simulink library "EasyGen3500_GensetSignalScaling_lib"  (Simulink 8.1)
settings: Solver=ode45  StartTime=0.0  StopTime=10.0  RelTol=1e-3
undefined symbols (not defined in the file): ph, Ts
libraries: rteventslib x4
settings Model: Creator=RE25624  LastModifiedBy=RE25624

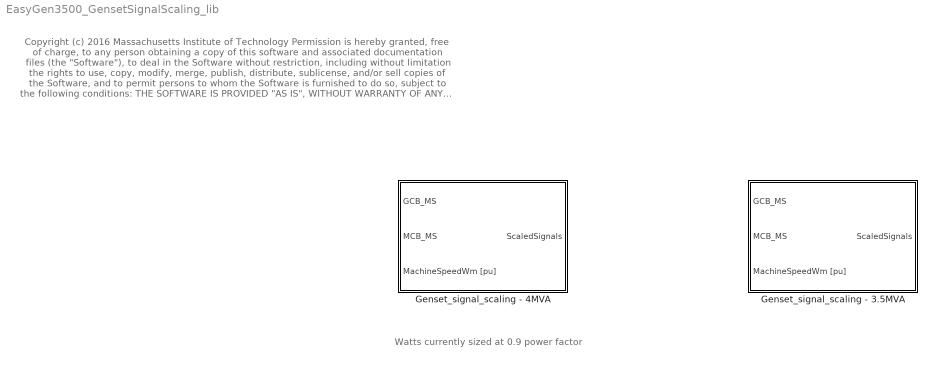
== system EasyGen3500_GensetSignalScaling_lib ==
  note: Watts currently sized at 0.9 power factor
  note: Copyright (c) 2016 Massachusetts Institute of Technology
      | Permission is hereby granted, free of charge, to any person obtaining a copy of this software and associated documentation files (the "Software"), to deal
      | in the Software without restriction, including without limitation the rights to use, copy, modify, merge, publish, distribute, sublicense, and/or sell copies of the
      | Software, and to permit persons to whom the Software is furnished to do so, subject to the following conditions:
      |
      | THE SOFTWARE IS PROVIDED "AS IS", WITHOUT WARRANTY OF ANY KIND, EXPRESS OR IMPLIED, INCLUDING BUT NOT LIMITED TO THE
      | WARRANTIES OF MERCHANTABILITY, FITNESS FOR A PARTICULAR PURPOSE AND NONINFRINGEMENT. IN NO EVENT SHALL THE AUTHORS
      | OR COPYRIGHT HOLDERS BE LIABLE FOR ANY CLAIM, DAMAGES OR OTHER LIABILITY, WHETHER IN AN ACTION OF CONTRACT, TORT OR
      | OTHERWISE, ARISING FROM, OUT OF OR IN CONNECTION WITH THE SOFTWARE OR THE USE OR OTHER DEALINGS IN THE SOFTWARE
  Genset_signal_scaling - 3.5MVA : Subsystem  mask(Genset Signal Scaling for Opal-RT/Woodward){Vpk_mcb=11268, watt_mcb=3150000, Vpk_gcb=11268, watt_gcb=3150000, rated_rpm=1800, wm_noise_bias=0.02}
      mask prompts: Vpk_mcb "MCB Nominal Voltage [Vpk]"; watt_mcb "MCB Watts [W]"; Vpk_gcb "GCB Nominal Voltage [ Vpk]"; watt_gcb "GCB Watts [W]"; rated_rpm "Machine Rated Speed [RPM]"; wm_noise_bias "Speed Noise Bias [0-1]"
      mask help:
      | Scaling for voltages:
      | For 120 => 12Vout / 170Vpk
      | For 480 => 12Vout / 391Vpk
      | For 13.8kv => 12Vout / 11268Vpk
      |
      | Scaling for currents - used in the 1 MVA genset:
      | 15Vout / ( 900000W / 391Vpk)
      |
      | Scaling for currents - used in the 3.5 MVA NG/CHP:
      | 15Vout / ( 3150000W / 11268Vpk)
      | - Current scale factors chosen to match easYgen settings for 3.5 MVA gas engine CT ratio of 1500/x made on 20160508
  Genset_signal_scaling - 4MVA : Subsystem  mask(Genset Signal Scaling for Opal-RT/Woodward){Vpk_mcb=11268, watt_mcb=3600000, Vpk_gcb=11268, watt_gcb=3600000, rated_rpm=1800, wm_noise_bias=0.02}
      mask prompts: Vpk_mcb "MCB Nominal Voltage [Vpk]"; watt_mcb "MCB Watts [W]"; Vpk_gcb "GCB Nominal Voltage [ Vpk]"; watt_gcb "GCB Watts [W]"; rated_rpm "Machine Rated Speed [RPM]"; wm_noise_bias "Speed Noise Bias [0-1]"
      mask help:
      | Scaling for voltages:
      | For 120 => 12Vout / 170Vpk
      | For 480 => 12Vout / 391Vpk
      | For 13.8kv => 12Vout / 11268Vpk
      |
      | Scaling for currents - used in the 1 MVA genset:
      | 15Vout / ( 900000W / 391Vpk)
      |
      | Scaling for currents - used in the 3.5 MVA NG/CHP:
      | 15Vout / ( 3150000W / 11268Vpk)
      | - Current scale factors chosen to match easYgen settings for 3.5 MVA gas engine CT ratio of 1500/x made on 20160508

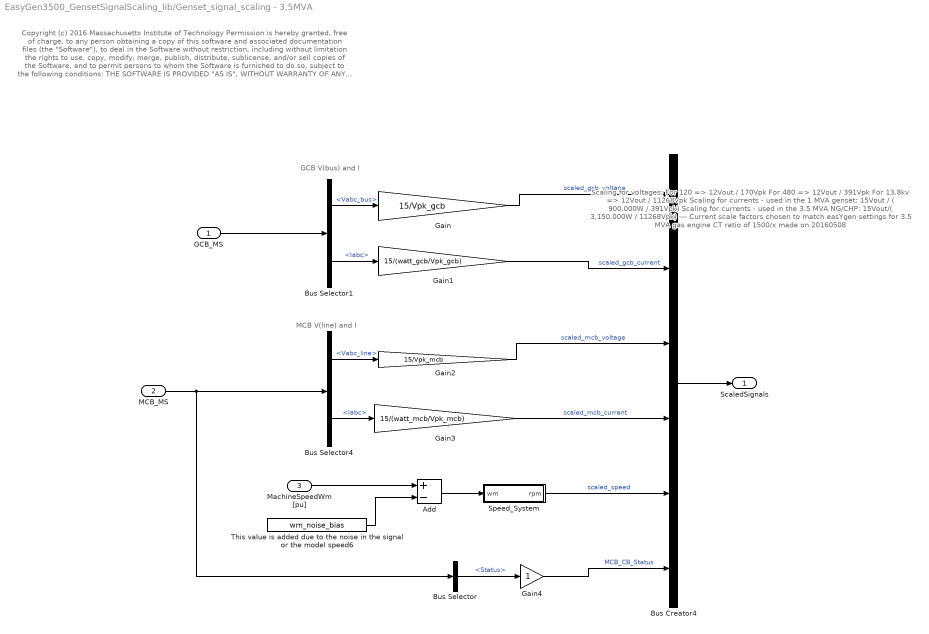
== system EasyGen3500_GensetSignalScaling_lib/Genset_signal_scaling - 3.5MVA ==
  note: Copyright (c) 2016 Massachusetts Institute of Technology
      | Permission is hereby granted, free of charge, to any person obtaining a copy of this software and associated documentation files (the "Software"), to deal
      | in the Software without restriction, including without limitation the rights to use, copy, modify, merge, publish, distribute, sublicense, and/or sell copies of the
      | Software, and to permit persons to whom the Software is furnished to do so, subject to the following conditions:
      |
      | THE SOFTWARE IS PROVIDED "AS IS", WITHOUT WARRANTY OF ANY KIND, EXPRESS OR IMPLIED, INCLUDING BUT NOT LIMITED TO THE
      | WARRANTIES OF MERCHANTABILITY, FITNESS FOR A PARTICULAR PURPOSE AND NONINFRINGEMENT. IN NO EVENT SHALL THE AUTHORS
      | OR COPYRIGHT HOLDERS BE LIABLE FOR ANY CLAIM, DAMAGES OR OTHER LIABILITY, WHETHER IN AN ACTION OF CONTRACT, TORT OR
      | OTHERWISE, ARISING FROM, OUT OF OR IN CONNECTION WITH THE SOFTWARE OR THE USE OR OTHER DEALINGS IN THE SOFTWARE
  note: Scaling for voltages:
      | For 120 => 12Vout / 170Vpk
      | For 480 => 12Vout / 391Vpk
      | For 13.8kv => 12Vout / 11268Vpk
      |
      | Scaling for currents - used in the 1 MVA genset:
      | 15Vout / ( 900,000W / 391Vpk)
      |
      | Scaling for currents - used in the 3.5 MVA NG/CHP:
      | 15Vout/( 3,150,000W / 11268Vpk)
      | --- Current scale factors chosen to match easYgen settings for 3.5 MVA gas engine CT ratio of 1500/x made on 20160508
  note: MCB V(line) and I
  note: GCB V(bus) and I
  GCB_MS : Inport
  MCB_MS : Inport  Port=2
  MachineSpeedWm [pu] : Inport  Port=3
  Add : Sum  Inputs=+-
  Bus Creator4 : BusCreator  Inputs=6
  Bus Selector : BusSelector  OutputSignals=Status
  Bus Selector1 : BusSelector  OutputSignals=Vabc_bus,Iabc
  Bus Selector4 : BusSelector  OutputSignals=Vabc_line,Iabc
  Gain : Gain  Gain=15/Vpk_gcb
  Gain1 : Gain  Gain=15/(watt_gcb/Vpk_gcb)
  Gain2 : Gain  Gain=15/Vpk_mcb
  Gain3 : Gain  Gain=15/(watt_mcb/Vpk_mcb)
  Gain4 : Gain
  Speed_System : Subsystem  mask{rated_rpm=rated_rpm}
      mask prompts: rated_rpm "Machine Rated Speed [RPM]"
  This value is added due to the noise in the signal or the model speed6 : Constant  Value=wm_noise_bias
  ScaledSignals : Outport
  wires:
  Bus Selector/1 -> Gain4/1  "<Status>"
  Gain4/1 -> Bus Creator4/6  "MCB_CB_Status"
  Gain/1 -> Bus Creator4/1  "scaled_gcb_voltage"
  Gain1/1 -> Bus Creator4/2  "scaled_gcb_current"
  Speed_System/1(rpm) -> Bus Creator4/5  "scaled_speed"
  Gain2/1 -> Bus Creator4/3  "scaled_mcb_voltage"
  Bus Creator4/1 -> ScaledSignals/1
  Bus Selector4/1 -> Gain2/1  "<Vabc_line>"
  Bus Selector4/2 -> Gain3/1  "<Iabc>"
  Gain3/1 -> Bus Creator4/4  "scaled_mcb_current"
  Bus Selector1/2 -> Gain1/1  "<Iabc>"
  Bus Selector1/1 -> Gain/1  "<Vabc_bus>"
  Add/1 -> Speed_System/1(wm)
  MCB_MS/1 -> Bus Selector/1, Bus Selector4/1
  GCB_MS/1 -> Bus Selector1/1
  MachineSpeedWm [pu]/1 -> Add/1
  This value is added due to the noise in the signal or the model speed6/1 -> Add/2

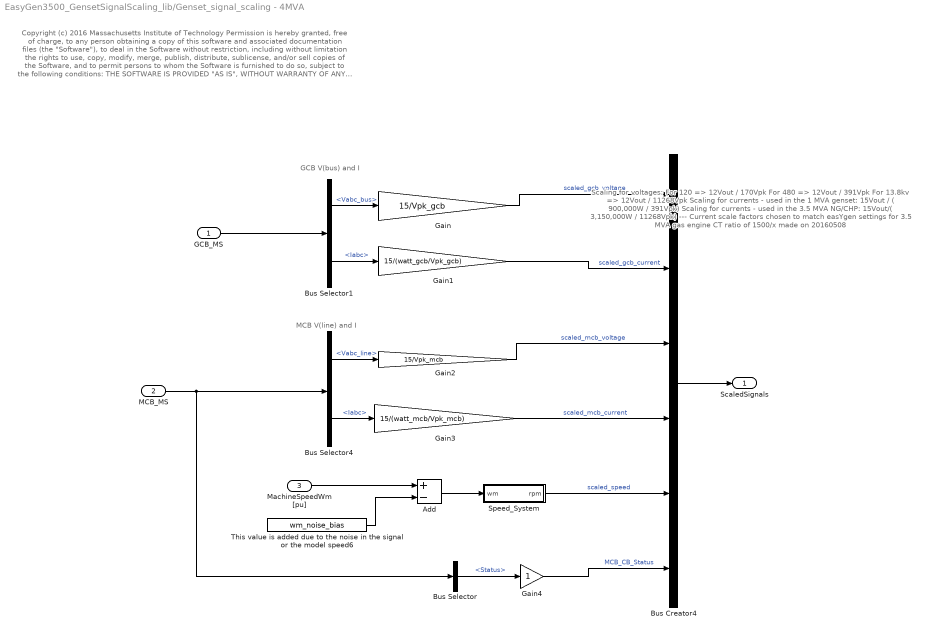
== system EasyGen3500_GensetSignalScaling_lib/Genset_signal_scaling - 4MVA ==
  note: GCB V(bus) and I
  note: MCB V(line) and I
  note: Scaling for voltages:
      | For 120 => 12Vout / 170Vpk
      | For 480 => 12Vout / 391Vpk
      | For 13.8kv => 12Vout / 11268Vpk
      |
      | Scaling for currents - used in the 1 MVA genset:
      | 15Vout / ( 900,000W / 391Vpk)
      |
      | Scaling for currents - used in the 3.5 MVA NG/CHP:
      | 15Vout/( 3,150,000W / 11268Vpk)
      | --- Current scale factors chosen to match easYgen settings for 3.5 MVA gas engine CT ratio of 1500/x made on 20160508
  note: Copyright (c) 2016 Massachusetts Institute of Technology
      | Permission is hereby granted, free of charge, to any person obtaining a copy of this software and associated documentation files (the "Software"), to deal
      | in the Software without restriction, including without limitation the rights to use, copy, modify, merge, publish, distribute, sublicense, and/or sell copies of the
      | Software, and to permit persons to whom the Software is furnished to do so, subject to the following conditions:
      |
      | THE SOFTWARE IS PROVIDED "AS IS", WITHOUT WARRANTY OF ANY KIND, EXPRESS OR IMPLIED, INCLUDING BUT NOT LIMITED TO THE
      | WARRANTIES OF MERCHANTABILITY, FITNESS FOR A PARTICULAR PURPOSE AND NONINFRINGEMENT. IN NO EVENT SHALL THE AUTHORS
      | OR COPYRIGHT HOLDERS BE LIABLE FOR ANY CLAIM, DAMAGES OR OTHER LIABILITY, WHETHER IN AN ACTION OF CONTRACT, TORT OR
      | OTHERWISE, ARISING FROM, OUT OF OR IN CONNECTION WITH THE SOFTWARE OR THE USE OR OTHER DEALINGS IN THE SOFTWARE
  GCB_MS : Inport
  MCB_MS : Inport  Port=2
  MachineSpeedWm [pu] : Inport  Port=3
  Add : Sum  Inputs=+-
  Bus Creator4 : BusCreator  Inputs=6
  Bus Selector : BusSelector  OutputSignals=Status
  Bus Selector1 : BusSelector  OutputSignals=Vabc_bus,Iabc
  Bus Selector4 : BusSelector  OutputSignals=Vabc_line,Iabc
  Gain : Gain  Gain=15/Vpk_gcb
  Gain1 : Gain  Gain=15/(watt_gcb/Vpk_gcb)
  Gain2 : Gain  Gain=15/Vpk_mcb
  Gain3 : Gain  Gain=15/(watt_mcb/Vpk_mcb)
  Gain4 : Gain
  Speed_System : Subsystem  mask{rated_rpm=rated_rpm}
      mask prompts: rated_rpm "Machine Rated Speed [RPM]"
  This value is added due to the noise in the signal or the model speed6 : Constant  Value=wm_noise_bias
  ScaledSignals : Outport
  wires:
  This value is added due to the noise in the signal or the model speed6/1 -> Add/2
  MachineSpeedWm [pu]/1 -> Add/1
  GCB_MS/1 -> Bus Selector1/1
  MCB_MS/1 -> Bus Selector4/1, Bus Selector/1
  Add/1 -> Speed_System/1(wm)
  Bus Selector1/1 -> Gain/1  "<Vabc_bus>"
  Bus Selector1/2 -> Gain1/1  "<Iabc>"
  Gain3/1 -> Bus Creator4/4  "scaled_mcb_current"
  Bus Selector4/2 -> Gain3/1  "<Iabc>"
  Bus Selector4/1 -> Gain2/1  "<Vabc_line>"
  Bus Creator4/1 -> ScaledSignals/1
  Gain2/1 -> Bus Creator4/3  "scaled_mcb_voltage"
  Speed_System/1(rpm) -> Bus Creator4/5  "scaled_speed"
  Gain1/1 -> Bus Creator4/2  "scaled_gcb_current"
  Gain/1 -> Bus Creator4/1  "scaled_gcb_voltage"
  Gain4/1 -> Bus Creator4/6  "MCB_CB_Status"
  Bus Selector/1 -> Gain4/1  "<Status>"

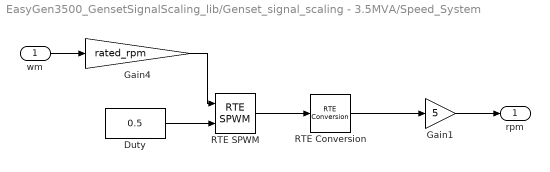
== system EasyGen3500_GensetSignalScaling_lib/Genset_signal_scaling - 3.5MVA/Speed_System ==
  wm : Inport
  Duty : Constant  DisableCoverage=on  Value=0.5
  Gain1 : Gain  Gain=5
  Gain4 : Gain  Gain=rated_rpm
  RTE Conversion : rteventslib/Signal Attributes/RTE Conversion  inputdatatype=RTE Boolean  outputdatatype=Double  compensation=Disabled  nbMaxEvents=10  sampleTime=Ts
  RTE SPWM : rteventslib/Sources/RTE SPWM  NumberPhases=1-ph  CenterAlignmentMode=On  MaxFreq=inf  MinFreq=0  EnablingPort=off  ComplementaryMode=off  SpaceVector=off  RiseTimeDelay=0  MaxEvents=10  SampleTime=Ts
  rpm : Outport
  wires:
  Gain4/1 -> RTE SPWM/1
  wm/1 -> Gain4/1
  RTE SPWM/1 -> RTE Conversion/1
  Duty/1 -> RTE SPWM/2
  RTE Conversion/1 -> Gain1/1
  Gain1/1 -> rpm/1

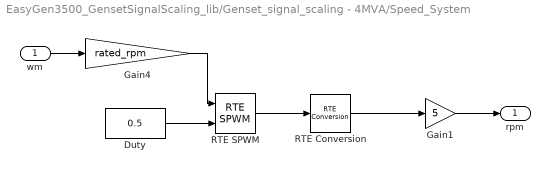
== system EasyGen3500_GensetSignalScaling_lib/Genset_signal_scaling - 4MVA/Speed_System ==
  wm : Inport
  Duty : Constant  DisableCoverage=on  Value=0.5
  Gain1 : Gain  Gain=5
  Gain4 : Gain  Gain=rated_rpm
  RTE Conversion : rteventslib/Signal Attributes/RTE Conversion  inputdatatype=RTE Boolean  outputdatatype=Double  compensation=Disabled  nbMaxEvents=10  sampleTime=Ts
  RTE SPWM : rteventslib/Sources/RTE SPWM  NumberPhases=1-ph  CenterAlignmentMode=On  MaxFreq=inf  MinFreq=0  EnablingPort=off  ComplementaryMode=off  SpaceVector=off  RiseTimeDelay=0  MaxEvents=10  SampleTime=Ts
  rpm : Outport
  wires:
  Gain1/1 -> rpm/1
  RTE Conversion/1 -> Gain1/1
  Duty/1 -> RTE SPWM/2
  RTE SPWM/1 -> RTE Conversion/1
  wm/1 -> Gain4/1
  Gain4/1 -> RTE SPWM/1
